simulink model "task_1_sim"  (R2023a)
settings: Solver=VariableStepAuto  StartTime=0.0  StopTime=15  MaxStep=1e-4  RelTol=1e-4
undefined symbols (not defined in the file): A, B, Bf, C, D, Df, G_f, G_g, K, Kf, Kg, w_f0, w_g0, x0, Y_f, Y_g
settings Model: Creator=user  LastModifiedBy=user

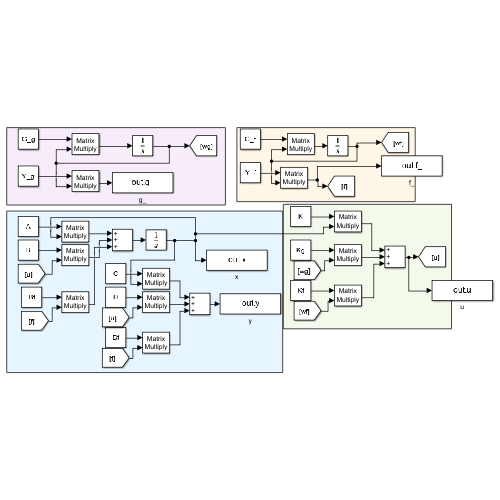
[thumbnail: Simulink's stored preview of the top-level diagram]
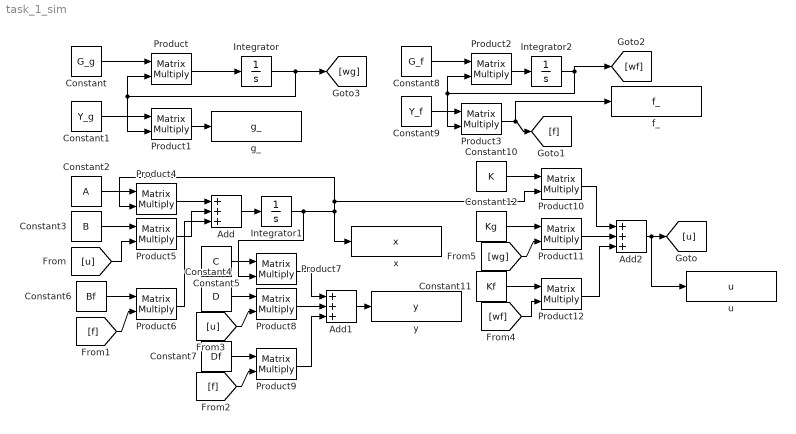
== system task_1_sim ==
  Add : Sum  Inputs=+++
  Add1 : Sum  Inputs=+++
  Add2 : Sum  Inputs=+++
  Constant : Constant  Value=G_g  VectorParams1D=off
  Constant1 : Constant  Value=Y_g  VectorParams1D=off
  Constant10 : Constant  Value=K  VectorParams1D=off
  Constant11 : Constant  Value=Kf  VectorParams1D=off
  Constant12 : Constant  Value=Kg  VectorParams1D=off
  Constant2 : Constant  Value=A  VectorParams1D=off
  Constant3 : Constant  Value=B  VectorParams1D=off
  Constant4 : Constant  Value=D  VectorParams1D=off
  Constant5 : Constant  Value=C  VectorParams1D=off
  Constant6 : Constant  Value=Bf  VectorParams1D=off
  Constant7 : Constant  Value=Df  VectorParams1D=off
  Constant8 : Constant  Value=G_f  VectorParams1D=off
  Constant9 : Constant  Value=Y_f  VectorParams1D=off
  Integrator : Integrator  InitialCondition=w_g0
  Integrator1 : Integrator  InitialCondition=x0
  Integrator2 : Integrator  InitialCondition=w_f0
  Product{,1..12} (13 alike) : Product  Multiplication=Matrix(*)
  f_ : ToWorkspace  VariableName=f_  SaveFormat=Timeseries  SampleTime=-1
  g_ : ToWorkspace  VariableName=g_  SaveFormat=Timeseries  SampleTime=-1
  u : ToWorkspace  VariableName=u  SaveFormat=Timeseries  SampleTime=-1
  x : ToWorkspace  VariableName=x  SaveFormat=Timeseries  SampleTime=-1
  y : ToWorkspace  VariableName=y  SaveFormat=Timeseries  SampleTime=-1
  wires:
  Constant/1 -> Product/1
  Product/1 -> Integrator/1
  Integrator/1 -> [wg], Product1/2, Product/2
  Constant1/1 -> Product1/1
  Product1/1 -> g_/1
  Constant8/1 -> Product2/1
  Product2/1 -> Integrator2/1
  Integrator2/1 -> [wf], Product3/2, Product2/2
  Constant9/1 -> Product3/1
  Product3/1 -> f_/1, [f]
  Constant2/1 -> Product4/1
  Integrator1/1 -> x/1, Product4/2, Product10/2, Product7/2
  Constant3/1 -> Product5/1
  [u] -> Product5/2
  Constant6/1 -> Product6/1
  [f] -> Product6/2
  Product4/1 -> Add/1
  Product5/1 -> Add/2
  Product6/1 -> Add/3
  Add/1 -> Integrator1/1
  Constant5/1 -> Product7/1
  Constant4/1 -> Product8/1
  [u] -> Product8/2
  Constant7/1 -> Product9/1
  [f] -> Product9/2
  Product7/1 -> Add1/1
  Product8/1 -> Add1/2
  Product9/1 -> Add1/3
  Add1/1 -> y/1
  Constant10/1 -> Product10/1
  Constant12/1 -> Product11/1
  [wg] -> Product11/2
  Constant11/1 -> Product12/1
  [wf] -> Product12/2
  Product10/1 -> Add2/1
  Product11/1 -> Add2/2
  Product12/1 -> Add2/3
  Add2/1 -> u/1, [u]
